simulink model "hoyas_grandes_i_2_sc_user_interface"  (R2023b)
settings: Solver=FixedStepDiscrete  StartTime=0.0  StopTime=inf  FixedStep=5e-05  RelTol=1e-3
PostLoadFcn:
  | Ts_Power=50e-6;f=50;R_ac=0.12;L_ac=0.08/(2*pi*50);L1=0.17874;L2=0.07596;L3=0.04321;L4=0.01471;L5=0.04751;L6=0.2054;L7=0.17263;L8=0.14418;L9=0.17697;L10=0.19944;L11=0.18905;L12=0.26987;L13=0.1671;L14=0.16874;L15=0.14664;L16=0.12477;L17=0.14989;L18=0.17217;L19=0.19436; load('PV_prof_norm.mat');
InitFcn:
  | Ts_Power=50e-6;f=50;R_ac=0.12;L_ac=0.08/(2*pi*50);L1=0.17874;L2=0.07596;L3=0.04321;L4=0.01471;L5=0.04751;L6=0.2054;L7=0.17263;L8=0.14418;L9=0.17697;L10=0.19944;L11=0.18905;L12=0.26987;L13=0.1671;L14=0.16874;L15=0.14664;L16=0.12477;L17=0.14989;L18=0.17217;L19=0.19436; load('PV_prof_norm.mat');
libraries: opal_lib x2
Description:
  | Model of a simple control system for use iin training.
settings Model: Creator=Paul Baracos  LastModifiedBy=depto
settings SolverCC: AlgebraicLoopSolver=TrustRegion
settings DataIOCC: LimitDataPoints=on  SaveFormat=Array  SignalLoggingSaveFormat=ModelDataLogs  SaveOutput=off  SaveTime=off  ReturnWorkspaceOutputs=off  SignalLoggingName=sigsOut
settings OptimizationCC: BlockReduction=off  BooleanDataType=off  OptimizeBlockIOStorage=off  BufferReuse=off  ExpressionFolding=off  LocalBlockOutputs=off  InitFltsAndDblsToZero=on  LifeSpan=inf
settings DebuggingCC: SaveWithParameterizedLinksMsg=none  UnderspecifiedInitializationDetection=Classic  MergeDetectMultiDrivingBlocksExec=none  SignalResolutionControl=TryResolveAllWithWarning  MultiTaskDSMMsg=warning  MultiTaskCondExecSysMsg=none  FcnCallInpInsideContextMsg=warning  UnconnectedInputMsg=warning  UnconnectedOutputMsg=warning  UnconnectedLineMsg=warning  SFUnexpectedBacktrackingDiag=warning  SFNoUnconditionalDefaultTransitionDiag=warning  SFExecutionAtInitializationDiag=none  ArithmeticOperatorsInVariantConditions=warning
settings HardwareCC: ProdBitPerPointer=32  ProdBitPerSizeT=32  ProdBitPerPtrDiffT=32  ProdLargestAtomicFloat=None  ProdIntDivRoundTo=Undefined  ProdEndianess=Unspecified  ProdWordSize=32  ProdHWDeviceType=32-bit Generic  TargetUnknown=on
settings ModelReferenceCC: EnableRefExpFcnMdlSchedulingChecks=on  PropagateSignalLabelsOutOfModel=off
settings SFSimCC: SimUseLocalCustomCode=off  CustomCodeUndefinedFunction=UseInterfaceOnly
settings RTWCC: GenCodeOnly=on  RTWUseLocalCustomCode=off
settings CodeAppCC: StateflowObjectComments=on
settings GRTTargetCC: TargetFcnLib=ansi_tfl_tmw.mat  TargetLangStandard=C89/C90 (ANSI)  CombineOutputUpdateFcns=off  GRTInterface=on
settings ConfigComp: CovMetricSettings=dw  CovSaveCumulativeToWorkspaceVar=on  CovSaveSingleToWorkspaceVar=on  CovExternalEMLEnable=off

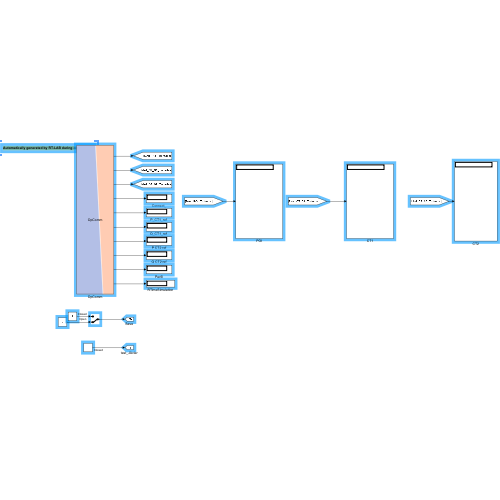
[thumbnail: Simulink's stored preview of the top-level diagram]
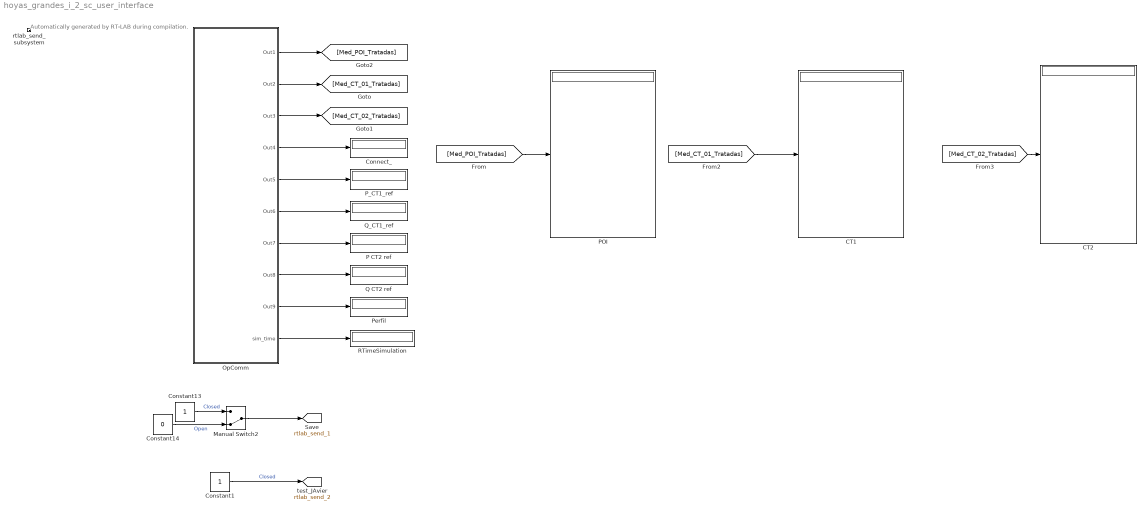
== system hoyas_grandes_i_2_sc_user_interface ==
  note: Automatically generated by RT-LAB during compilation.
  CT1 : Display
  CT2 : Display
  Connect_ : Display
  Constant1 : Constant
  Constant13 : Constant
  Constant14 : Constant  Value=0
  Manual Switch2 : ManualSwitch  CurrentSetting=0
  OpComm : Subsystem
      mask init:
      | opmaskdisplay('maskdisplay_block',gcb,'disp(''OpComm'')');
      mask Display:
      | patch([0 0.5 0.7 0],[1 1 0 0],[0.7 0.75 0.9]);
      | patch([1 0.53 0.73 1],[1 1 0 0],[1 0.8 0.7]);
      | plot([0 0 1 1 0],[0 1 1 0 0]);
      | disp('OpComm')
  P CT2 ref : Display
  POI : Display
  "P_CT1_ref " : Display
  Perfil : Display
  Q CT2 ref : Display
  "Q_CT1_ref " : Display
  RTimeSimulation : Display
  rtlab_send_subsystem : Subsystem  Priority=-100
      mask Display: text(0,0,'');
  tag scope: rtlab_send_1=global, rtlab_send_2=global
  wires:
  Constant1/1 -> [rtlab_send_2]  "Closed"
  [Med_CT_02_Tratadas] -> CT2/1
  [Med_POI_Tratadas] -> POI/1
  [Med_CT_01_Tratadas] -> CT1/1
  OpComm/1(Out1) -> [Med_POI_Tratadas]
  OpComm/3(Out3) -> [Med_CT_02_Tratadas]
  OpComm/2(Out2) -> [Med_CT_01_Tratadas]
  OpComm/4(Out4) -> Connect_/1
  OpComm/5(Out5) -> "P_CT1_ref "/1
  OpComm/6(Out6) -> "Q_CT1_ref "/1
  OpComm/7(Out7) -> P CT2 ref/1
  OpComm/9(Out9) -> Perfil/1
  OpComm/8(Out8) -> Q CT2 ref/1
  OpComm/10(sim_time) -> RTimeSimulation/1
  Constant13/1 -> Manual Switch2/1  "Closed"
  Manual Switch2/1 -> [rtlab_send_1]
  Constant14/1 -> Manual Switch2/2  "Open"

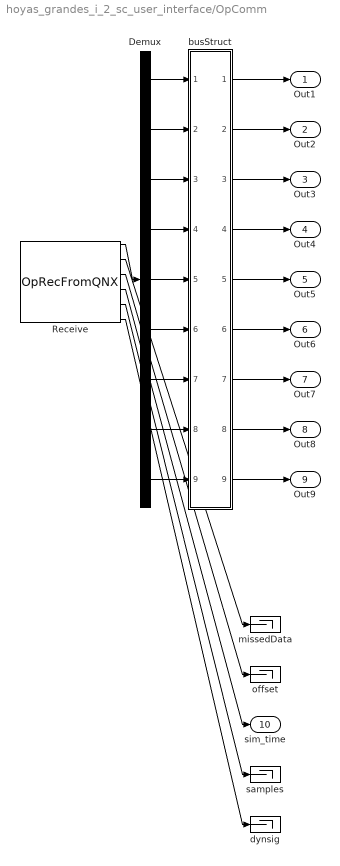
== system hoyas_grandes_i_2_sc_user_interface/OpComm ==
  Demux : Demux  Outputs="[12   8   8   1   1   1   1   1   1]"
  Receive : opal_lib/Communication/OpRecFromQNX  Node_num=1  Acqu_Group=1  Data_Width=34  Synchronization=on  Interpolation=on  Threshold=0.01  modelname=HOYAS_GRANDES_I  sampletime=5e-05
  busStruct : Subsystem
  dynsig : Terminator
  missedData : Terminator
  offset : Terminator
  samples : Terminator
  Out1 : Outport
  Out2 : Outport  Port=2
  Out3 : Outport  Port=3
  Out4 : Outport  Port=4
  Out5 : Outport  Port=5
  Out6 : Outport  Port=6
  Out7 : Outport  Port=7
  Out8 : Outport  Port=8
  Out9 : Outport  Port=9
  sim_time : Outport  Port=10
  wires:
  Demux/9 -> busStruct/9(In9)
  Demux/8 -> busStruct/8(In8)
  Demux/7 -> busStruct/7(In7)
  Demux/6 -> busStruct/6(In6)
  Demux/5 -> busStruct/5(In5)
  Demux/4 -> busStruct/4(In4)
  Demux/3 -> busStruct/3(In3)
  Demux/2 -> busStruct/2(In2)
  Demux/1 -> busStruct/1(In1)
  busStruct/9(Out9) -> Out9/1
  busStruct/8(Out8) -> Out8/1
  busStruct/7(Out7) -> Out7/1
  busStruct/6(Out6) -> Out6/1
  busStruct/5(Out5) -> Out5/1
  busStruct/4(Out4) -> Out4/1
  busStruct/3(Out3) -> Out3/1
  busStruct/2(Out2) -> Out2/1
  busStruct/1(Out1) -> Out1/1
  Receive/1 -> Demux/1
  Receive/6 -> dynsig/1
  Receive/5 -> samples/1
  Receive/4 -> sim_time/1
  Receive/3 -> offset/1
  Receive/2 -> missedData/1

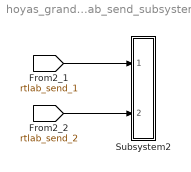
== system hoyas_grandes_i_2_sc_user_interface/rtlab_send_subsystem ==
  Subsystem2 : Subsystem
  wires:
  [rtlab_send_1] -> Subsystem2/1(In1)
  [rtlab_send_2] -> Subsystem2/2(In2)

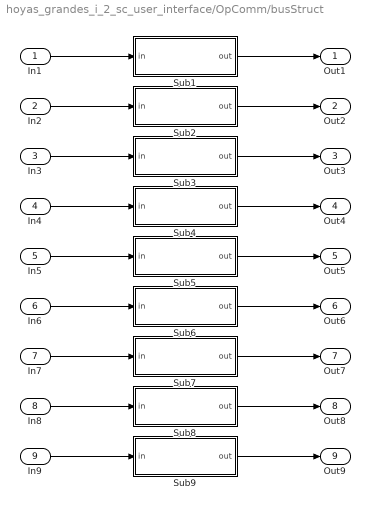
== system hoyas_grandes_i_2_sc_user_interface/OpComm/busStruct ==
  In1 : Inport
  In2 : Inport  Port=2
  In3 : Inport  Port=3
  In4 : Inport  Port=4
  In5 : Inport  Port=5
  In6 : Inport  Port=6
  In7 : Inport  Port=7
  In8 : Inport  Port=8
  In9 : Inport  Port=9
  Sub1 : Subsystem
  Sub2 : Subsystem
  Sub3 : Subsystem
  Sub4 : Subsystem
  Sub5 : Subsystem
  Sub6 : Subsystem
  Sub7 : Subsystem
  Sub8 : Subsystem
  Sub9 : Subsystem
  Out1 : Outport
  Out2 : Outport  Port=2
  Out3 : Outport  Port=3
  Out4 : Outport  Port=4
  Out5 : Outport  Port=5
  Out6 : Outport  Port=6
  Out7 : Outport  Port=7
  Out8 : Outport  Port=8
  Out9 : Outport  Port=9
  wires:
  Sub9/1(out) -> Out9/1
  In9/1 -> Sub9/1(in)
  Sub8/1(out) -> Out8/1
  In8/1 -> Sub8/1(in)
  Sub7/1(out) -> Out7/1
  In7/1 -> Sub7/1(in)
  Sub6/1(out) -> Out6/1
  In6/1 -> Sub6/1(in)
  Sub5/1(out) -> Out5/1
  In5/1 -> Sub5/1(in)
  Sub4/1(out) -> Out4/1
  In4/1 -> Sub4/1(in)
  Sub3/1(out) -> Out3/1
  In3/1 -> Sub3/1(in)
  Sub2/1(out) -> Out2/1
  In2/1 -> Sub2/1(in)
  Sub1/1(out) -> Out1/1
  In1/1 -> Sub1/1(in)

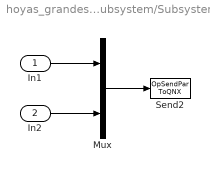
== system hoyas_grandes_i_2_sc_user_interface/rtlab_send_subsystem/Subsystem2 ==
  In1 : Inport  PortDimensions=1
  In2 : Inport  Port=2  PortDimensions=1
  Mux : Mux  Inputs=2
  Send2 : opal_lib/Communication/OpSendPar ToQNX  Node_num=1  modelname=HOYAS_GRANDES_I
  wires:
  Mux/1 -> Send2/1
  In1/1 -> Mux/1
  In2/1 -> Mux/2

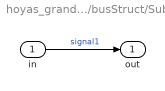
== system hoyas_grandes_i_2_sc_user_interface/OpComm/busStruct/Sub1 ==
  in : Inport
  out : Outport
  wires:
  in/1 -> out/1  "signal1"

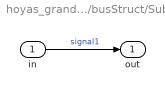
== system hoyas_grandes_i_2_sc_user_interface/OpComm/busStruct/Sub2 ==
  in : Inport
  out : Outport
  wires:
  in/1 -> out/1  "signal1"

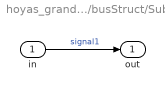
== system hoyas_grandes_i_2_sc_user_interface/OpComm/busStruct/Sub3 ==
  in : Inport
  out : Outport
  wires:
  in/1 -> out/1  "signal1"

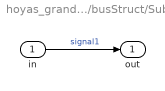
== system hoyas_grandes_i_2_sc_user_interface/OpComm/busStruct/Sub4 ==
  in : Inport
  out : Outport
  wires:
  in/1 -> out/1  "signal1"

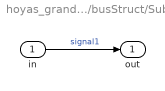
== system hoyas_grandes_i_2_sc_user_interface/OpComm/busStruct/Sub5 ==
  in : Inport
  out : Outport
  wires:
  in/1 -> out/1  "signal1"

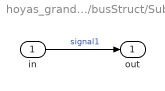
== system hoyas_grandes_i_2_sc_user_interface/OpComm/busStruct/Sub6 ==
  in : Inport
  out : Outport
  wires:
  in/1 -> out/1  "signal1"

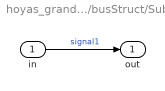
== system hoyas_grandes_i_2_sc_user_interface/OpComm/busStruct/Sub7 ==
  in : Inport
  out : Outport
  wires:
  in/1 -> out/1  "signal1"

== system hoyas_grandes_i_2_sc_user_interface/OpComm/busStruct/Sub8 ==
  in : Inport
  out : Outport
  wires:
  in/1 -> out/1  "signal1"

== system hoyas_grandes_i_2_sc_user_interface/OpComm/busStruct/Sub9 ==
  in : Inport
  out : Outport
  wires:
  in/1 -> out/1  "Data"
